simulink model "mass_sim"  (R2015a)
settings: Solver=ode45  StartTime=0.0  StopTime=100  RelTol=1e-3
InitFcn:
  | param
undefined symbols (not defined in the file or in its folder): drawMSD, mass_ctrl, P
settings Model: Creator=beard  LastModifiedBy=beard
settings DataIOCC: SignalLoggingSaveFormat=ModelDataLogs
settings OptimizationCC: ExpressionDepthLimit=2147483647  InitFltsAndDblsToZero=on
settings DebuggingCC: UnderspecifiedInitializationDetection=Classic  MergeDetectMultiDrivingBlocksExec=none  SolverPrmCheckMsg=warning  FcnCallInpInsideContextMsg=UseLocalSettings  StateNameClashWarn=warning
settings GRTTargetCC: CombineOutputUpdateFcns=off  GRTInterface=on

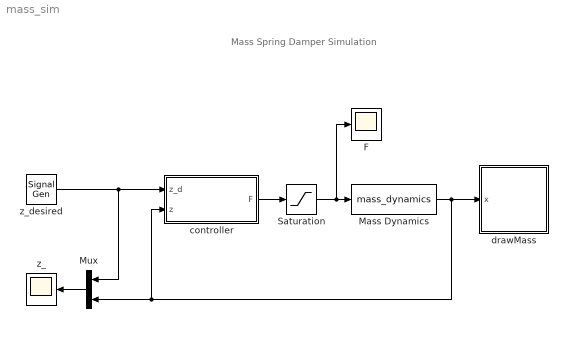
== system mass_sim ==
  note: Mass Spring Damper Simulation
  F : Scope
      settings: TimeRange=100  YMin=-1.75  YMax=2
  Mass Dynamics : S-Function  FunctionName=mass_dynamics  Parameters=AP
  Mux : Mux  Inputs=2
  Saturation : Saturate  UpperLimit=P.Fmax  LowerLimit=-P.Fmax
  controller : Subsystem
  drawMass : Subsystem
      mask Display: image(imread('tv.jpg'))
  z_ : Scope
      settings: TimeRange=100  YMin=-2  YMax=1.5
  z_desired : SignalGenerator  WaveForm=square  Amplitude=.5  Frequency=.01
  wires:
  z_desired/1 -> Mux/1, controller/1(z_d)
  Mass Dynamics/1 -> controller/2(z), Mux/2, drawMass/1(x)
  Mux/1 -> z_/1
  Saturation/1 -> F/1, Mass Dynamics/1
  controller/1(F) -> Saturation/1

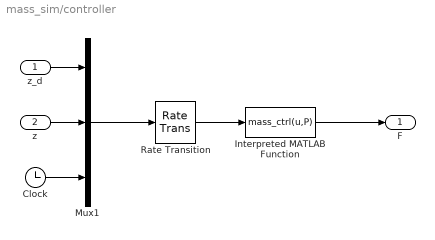
== system mass_sim/controller ==
  z_d : Inport
  z : Inport  Port=2
  Clock : Clock
  Interpreted MATLAB Function : MATLABFcn  MATLABFcn=mass_ctrl(u,P)  OutputDimensions=1
  Mux1 : Mux  Inputs=3
  Rate Transition : RateTransition  OutPortSampleTime=P.Ts
  F : Outport
  wires:
  Mux1/1 -> Rate Transition/1
  z_d/1 -> Mux1/1
  z/1 -> Mux1/2
  Interpreted MATLAB Function/1 -> F/1
  Clock/1 -> Mux1/3
  Rate Transition/1 -> Interpreted MATLAB Function/1

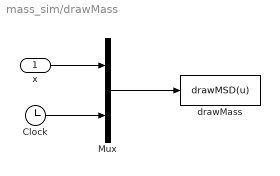
== system mass_sim/drawMass ==
  x : Inport
  Clock : Clock
  Mux : Mux  Inputs=2
  drawMass : MATLABFcn  MATLABFcn=drawMSD(u)  OutputDimensions=0  SampleTime=0.1
  wires:
  Clock/1 -> Mux/2
  x/1 -> Mux/1
  Mux/1 -> drawMass/1
